simulink model "controlled_source"  (R2015b)
settings: Solver=ode1  SolverMode=SingleTasking  StartTime=0.0  StopTime=10.0  FixedStep=Time_Step  MaxStep=50e-6  RelTol=1e-3
undefined symbols (not defined in the file): fb, L, R, Theta0, Time_Step, Ug
libraries: powerlib x8, spsPower3phInstantaneousLib x1
settings Model: Creator=Frederic_Colas  LastModifiedBy=Frederic_Colas
settings DataIOCC: LimitDataPoints=off  ReturnWorkspaceOutputs=on
settings DebuggingCC: AllowSymbolicDim=on  SFUnexpectedBacktrackingDiag=error  SFNoUnconditionalDefaultTransitionDiag=error
settings ModelReferenceCC: PropagateSignalLabelsOutOfModel=on
settings SFSimCC: SimUseLocalCustomCode=on
settings RTWCC: RTWUseLocalCustomCode=on
settings GRTTargetCC: TargetLangStandard=C99 (ISO)
settings ConfigComp: CovMetricSettings=dwe  CovSaveCumulativeToWorkspaceVar=off  CovSaveSingleToWorkspaceVar=off  CovModelRefEnable=Off  CovExternalEMLEnable=on

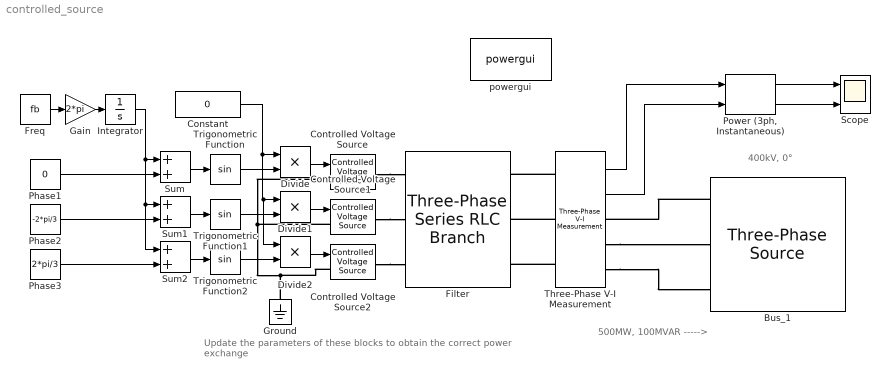
== system controlled_source ==
  note: 500MW, 100MVAR
      | ----->
  note: 400kV, 0°
  note: Update the parameters of these blocks
      | to obtain the correct power exchange
  Bus_1 : powerlib/Electrical Sources/Three-Phase Source  InternalConnection=Yg  VoltagePhases=off  Voltage=Ug  PhaseAngle=0  Voltage_phases=[25e3 25e3 25e3]/sqrt(3)  PhaseAngles_phases=[0 -120 +120]  Frequency=fb  NonIdealSource=off  SpecifyImpedance=off  Resistance=0.8929  Inductance=16.58e-3  ShortCircuitLevel=100e6  BaseVoltage=25e3  XRratio=7  BusType=swing  Pref=10e3  Qref=0  Prefabc=[10e3, 10e3, 10e3]  Qrefabc=[0, 0, 0]  Qmin=-inf  Qmax=inf
  Constant : Constant  Value=0
  Controlled Voltage Source : powerlib/Electrical Sources/Controlled Voltage Source  Initialize=on  Source_Type=AC  Amplitude=0  Phase=0  Frequency=fb  Measurements=None
  Controlled Voltage Source1 : powerlib/Electrical Sources/Controlled Voltage Source  Initialize=on  Source_Type=AC  Amplitude=0  Phase=0  Frequency=fb  Measurements=None
  Controlled Voltage Source2 : powerlib/Electrical Sources/Controlled Voltage Source  Initialize=on  Source_Type=AC  Amplitude=0  Phase=0  Frequency=fb  Measurements=None
  Divide : Product  Inputs=**
  Divide1 : Product  Inputs=**
  Divide2 : Product  Inputs=**
  Filter : powerlib/Elements/Three-Phase Series RLC Branch  LConnTagsString=A|B|C  RConnTagsString=A|B|C  BranchType=RL  Resistance=R  Inductance=L  Capacitance=1e-6  Measurements=None
  Freq : Constant  Value=fb
  Gain : Gain  Gain=2*pi
  Ground : powerlib/Elements/Ground  LConnTagsString=a
  Integrator : Integrator  InitialCondition=Theta0*pi/180
  Phase1 : Constant  Value=0
  Phase2 : Constant  Value=-2*pi/3
  Phase3 : Constant  Value=2*pi/3
  "Power (3ph, Instantaneous)" : spsPower3phInstantaneousLib/Power (3ph, Instantaneous)
  Scope : Scope  NumInputPorts=2
  Sum : Sum
  Sum1 : Sum
  Sum2 : Sum
  Three-Phase V-I Measurement : powerlib/Measurements/Three-Phase V-I Measurement  VoltageMeasurement=phase-to-ground  SetLabelV=off  LabelV=Vabc  Vpu=off  VpuLL=off  CurrentMeasurement=yes  SetLabelI=off  LabelI=Iabc  Ipu=off  Pbase=100e6  Vbase=500e3  OutputType=Complex  PhasorSimulation=off  PSBequivalent=0
  Trigonometric Function : Trigonometry
  Trigonometric Function1 : Trigonometry
  Trigonometric Function2 : Trigonometry
  powergui : powerlib/powergui  Priority=1  SimulationMode=Discrete  SampleTime=Time_Step  frequency=60  Iterations=50  frequencyindice=50  Pbase=1000000000  ErrMax=1e-6  UnitsV=kV  UnitsW=MW  buscounter=0  FunctionMessages=off  echomessages=off  EnableUseOfTLC=off  CurrentSourceSwitches=off  DisableSnubberDevices=off  DisableRonSwitches=off  DisableVfSwitches=off  DisplayEquations=off  AutomaticDiscreteSolvers=off  SolverType=Tustin/Backward Euler (TBE)  Interpol=off  ExternalGateDelay=off  methode=off  Ts=100  x0status=blocks  SPID=on  SwTol=0  HookPort=off  NonlinearTolerance=1e-4  nMaxIteration=100  ContinueOnMaxIteration=off  RestoreLinks=warning  ResistiveCurrentMeasurement=off  Frange=[0:2:500]  Ylog=off  Xlog=on  ShowGrid=off  save=off  variable=ZData  structure=0  ZoomFFT=off  StartTime=0.0  cycles=1  DisplayStyle=1  fundamental=60  FreqAxis=off  MaxFrequency=1000  frequencyindicesteady=1  RmsSteady=1  display=off
  wires:
  Three-Phase V-I Measurement/1 -> "Power (3ph, Instantaneous)"/1
  Three-Phase V-I Measurement/2 -> "Power (3ph, Instantaneous)"/2
  "Power (3ph, Instantaneous)"/1 -> Scope/1
  "Power (3ph, Instantaneous)"/2 -> Scope/2
  Trigonometric Function/1 -> Divide/2
  Trigonometric Function1/1 -> Divide1/2
  Trigonometric Function2/1 -> Divide2/2
  Sum/1 -> Trigonometric Function/1
  Phase1/1 -> Sum/2
  Sum1/1 -> Trigonometric Function1/1
  Phase2/1 -> Sum1/2
  Sum2/1 -> Trigonometric Function2/1
  Phase3/1 -> Sum2/2
  Freq/1 -> Gain/1
  Integrator/1 -> Sum2/1, Sum1/1, Sum/1
  Divide/1 -> Controlled Voltage Source/1
  Divide1/1 -> Controlled Voltage Source1/1
  Divide2/1 -> Controlled Voltage Source2/1
  Constant/1 -> Divide2/1, Divide1/1, Divide/1
  Gain/1 -> Integrator/1
  connections:
  Three-Phase V-I Measurement/LConn1 -- Filter/RConn1
  Three-Phase V-I Measurement/LConn2 -- Filter/RConn2
  Three-Phase V-I Measurement/LConn3 -- Filter/RConn3
  Bus_1/RConn1 -- Three-Phase V-I Measurement/RConn1
  Three-Phase V-I Measurement/RConn2 -- Bus_1/RConn2
  Three-Phase V-I Measurement/RConn3 -- Bus_1/RConn3
  Controlled Voltage Source/RConn1 -- Filter/LConn1
  Controlled Voltage Source1/RConn1 -- Filter/LConn2
  Controlled Voltage Source2/RConn1 -- Filter/LConn3
  Controlled Voltage Source/LConn1 -- Controlled Voltage Source1/LConn1 -- Controlled Voltage Source2/LConn1 -- Ground/LConn1
